simulink model "Ejercicio_3"  (R2013a)
settings: Solver=ode45  StartTime=0.0  StopTime=20  RelTol=1e-3
settings Model: Creator=Miguel  LastModifiedBy=Miguel

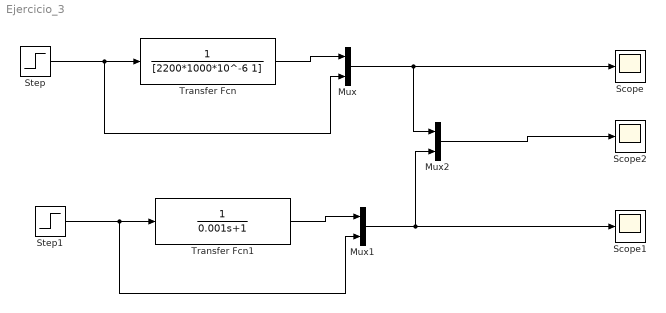
== system Ejercicio_3 ==
  Mux : Mux  Inputs=2
  Mux1 : Mux  Inputs=2
  Mux2 : Mux  Inputs=2
  Scope : Scope
  Scope1 : Scope
  Scope2 : Scope
      settings: SaveName=ScopeData2
  Step : Step  SampleTime=0
  Step1 : Step  SampleTime=0
  Transfer Fcn : TransferFcn  Denominator=[2200*1000*10^-6 1]
  Transfer Fcn1 : TransferFcn  Denominator=[0.001 1]
  wires:
  Mux/1 -> Mux2/1, Scope/1
  Step/1 -> Mux/2, Transfer Fcn/1
  Transfer Fcn/1 -> Mux/1
  Mux1/1 -> Mux2/2, Scope1/1
  Step1/1 -> Mux1/2, Transfer Fcn1/1
  Transfer Fcn1/1 -> Mux1/1
  Mux2/1 -> Scope2/1
